simulink model "Crane_LQR_disc_Kalman"  (R2018a)
settings: Solver=VariableStepAuto  StartTime=0.0  StopTime=30  RelTol=1e-3
undefined symbols (not defined in the file): A, B, C, D, Discrete, F, L, sigbuilder_block, Time, Ts, xinit
libraries: dspsrcs4 x1, ctrlSharedLib x1
settings Model: Creator=tcbooij  LastModifiedBy=TU Delf SID
settings CodeAppCC: StateflowObjectComments=on

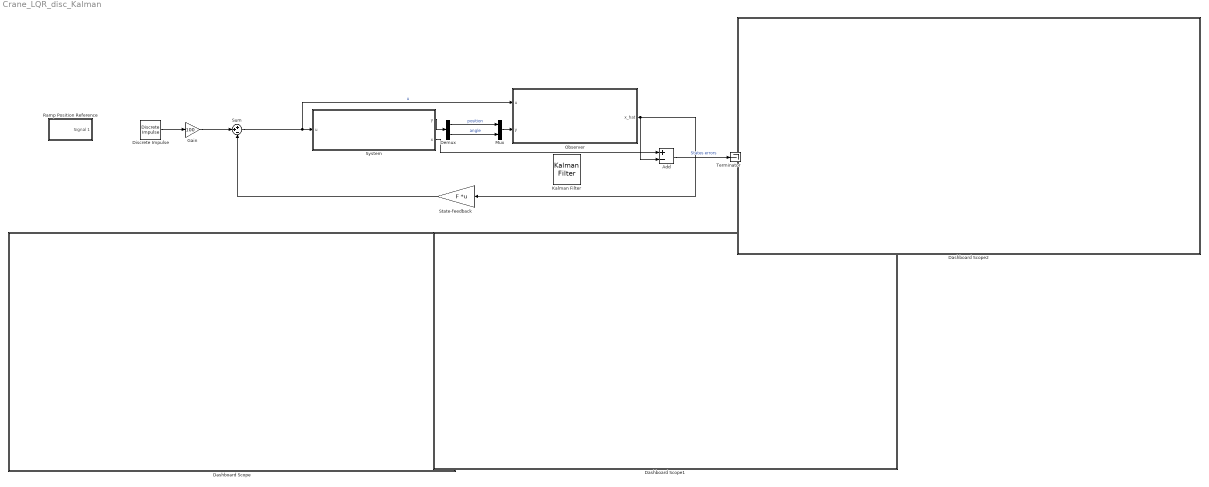
== system Crane_LQR_disc_Kalman ==
  Add : Sum  Inputs=+-
  Dashboard Scope : Subsystem  DialogController=hmiCreateDDGDialog  IsWebBlock=on  mask(MWDashboardBlock){webBlockId=2d634a0c-9c30-41ca-882d-9c1a5de680b0, webBlockType=sdiscope, ShowInitialText=on, HMISrcModelName=Crane_LQR_disc2}
      mask prompts: webBlockId "WebBlock Id"; webBlockType "WebBlock Type"; HMISrcModelName "Source Model"
      mask help: SimulinkHMI:dialogs:HMIScopeDialogDesc
      mask Help: helpview([docroot '/mapfiles/simulink.map'], 'hmi_scope')
      mask Display:
      | if strcmp(get_param(bdroot(gcb),'BlockDiagramType'), 'library')
      |     image([(matlabroot) '/toolbox/simulink/hmi/icons/DashboardScope.png']);
      | end
  Dashboard Scope1 : Subsystem  DialogController=hmiCreateDDGDialog  IsWebBlock=on  mask(MWDashboardBlock){webBlockId=94ce42f8-c4e1-41da-82c1-a31c02963333, webBlockType=sdiscope, ShowInitialText=on, HMISrcModelName=Crane_LQR_disc2}
      mask prompts: webBlockId "WebBlock Id"; webBlockType "WebBlock Type"; HMISrcModelName "Source Model"
      mask help: SimulinkHMI:dialogs:HMIScopeDialogDesc
      mask Help: helpview([docroot '/mapfiles/simulink.map'], 'hmi_scope')
      mask Display:
      | if strcmp(get_param(bdroot(gcb),'BlockDiagramType'), 'library')
      |     image([(matlabroot) '/toolbox/simulink/hmi/icons/DashboardScope.png']);
      | end
  Dashboard Scope2 : Subsystem  DialogController=hmiCreateDDGDialog  IsWebBlock=on  mask(MWDashboardBlock){webBlockId=eee89b98-8c9a-4aeb-b6f7-67e202be8cd2, webBlockType=sdiscope, ShowInitialText=on, HMISrcModelName=Crane_LQR_disc2}
      mask prompts: webBlockId "WebBlock Id"; webBlockType "WebBlock Type"; HMISrcModelName "Source Model"
      mask help: SimulinkHMI:dialogs:HMIScopeDialogDesc
      mask Help: helpview([docroot '/mapfiles/simulink.map'], 'hmi_scope')
      mask Display:
      | if strcmp(get_param(bdroot(gcb),'BlockDiagramType'), 'library')
      |     image([(matlabroot) '/toolbox/simulink/hmi/icons/DashboardScope.png']);
      | end
  Demux : Demux  Outputs=2
  Discrete Impulse : dspsrcs4/Discrete  Impulse  Delay=200  SampleTime=0.01  FrameSample=1  OutputFrames=off  dataType=double  isSigned=on  wordLen=16  udDataType=sfix(16)  fracBitsMode=Best precision  numFracBits=15  OutDataTypeStr=double  LastOutDataTypeStr=double
  Gain : Gain  Gain=100
  Kalman Filter : ctrlSharedLib/Kalman Filter  TimeDomain=Discrete-Time  UseCurrentEstimator=on  ModelSource=Individual A, B, C, D matrices  ModelSourceVariable=ss(A,B,C,D,Ts)  A=A  B=B  C=C  D=D  NumberOfStates=1  NumberOfInputs=1  NumberOfOutputs=1  InitialEstimateSource=Dialog  X0=0  P0=10  UseK=off  UseGH=off  NumberOfProcessNoiseInputs=1  G=1  TimeInvariantG=on  H=0  TimeInvariantH=on  Q=0.05  TimeInvariantQ=on  R=1  TimeInvariantR=on  N=0  TimeInvariantN=on  AddInputPort=on  AddEnablePort=off  OutputEstimatedY=off  OutputP=off  Ts=-1
      settings: SourceProductBaseCode=CT
  Mux : Mux  Inputs=2
  Observer : Subsystem
  Ramp Position Reference : Subsystem  Tag=STV Subsys  LoadFcn=sigbuilder_block('load');  StartFcn=sigbuilder_block('start');  StopFcn=sigbuilder_block('stop');  ClipboardFcn=sigbuilder_block('clipboard');  mask(Sigbuilder block){tuvar=[0:10]}
      mask help: Simulink:masks:SigbuilderBlock_MD
      mask init:
      | if ~strcmp(get_param(bdroot(gcbh),'SimulationStatus'),'stopped') tuvar = sigbuilder_block('maskInit'); end
      settings: CopyFcn=sigbuilder_block('copy');  DeleteFcn=sigbuilder_block('delete');  ModelCloseFcn=sigbuilder_block('modelClose');  PreSaveFcn=sigbuilder_block('preSave');  PauseFcn=sigbuilder_block('pause');  ContinueFcn=sigbuilder_block('continue');  NameChangeFcn=sigbuilder_block('namechange');  OpenFcn=sigbuilder_block('open',[294 84 558 400.5 ]);  CloseFcn=sigbuilder_block('close');
      mask Display: plot(0, 0, 100, 100,[2, 2, 32, 32, 2], [68, 8, 8, 68, 68],[32, 2], [38, 38], [32, 19, 2],[53, 60, 44], [32, 17, 17, 2],[16, 16, 31, 31]);txt = getActiveGroup(gcbh);text(2, 100, txt,'verticalAlignment', 'top');
  State-feedback : Gain  Gain=F  Multiplication=Matrix(K*u)
  Sum : Sum  Inputs=++-
  System : Subsystem
  Terminator : Terminator
  wires:
  Sum/1 -> Observer/1(u), System/1(u)  "u"
  State-feedback/1 -> Sum/3
  Observer/1(x_hat) -> Add/2, State-feedback/1
  System/1(y) -> Demux/1
  Mux/1 -> Observer/2(y)
  Demux/1 -> Mux/1  "position"
  Demux/2 -> Mux/2  "angle"
  Discrete Impulse/1 -> Gain/1
  Gain/1 -> Sum/2
  System/2(x) -> Add/1
  Add/1 -> Terminator/1  "States errors"

== system Crane_LQR_disc_Kalman/Dashboard Scope ==

== system Crane_LQR_disc_Kalman/Dashboard Scope1 ==

== system Crane_LQR_disc_Kalman/Dashboard Scope2 ==

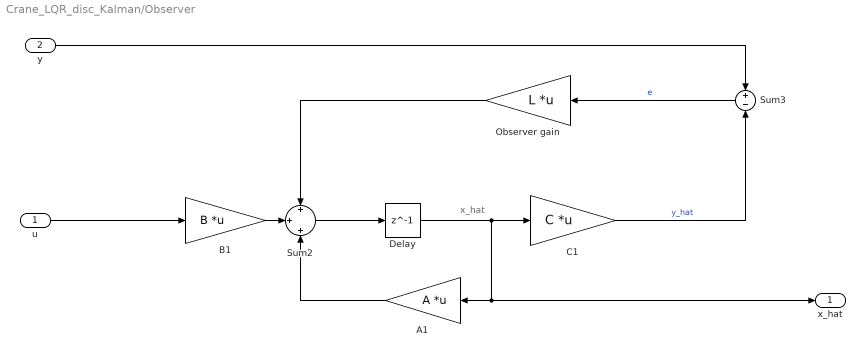
== system Crane_LQR_disc_Kalman/Observer ==
  note: x_hat
  u : Inport
  y : Inport  Port=2
  A1 : Gain  Gain=A  Multiplication=Matrix(K*u)
  B1 : Gain  Gain=B  Multiplication=Matrix(K*u)
  C1 : Gain  Gain=C  Multiplication=Matrix(K*u)
  Delay : Delay  DelayLength=1
  Observer gain : Gain  Gain=L  Multiplication=Matrix(K*u)
  Sum2 : Sum  Inputs=+|+|+
  Sum3 : Sum  Inputs=+|-
  x_hat : Outport
  wires:
  Sum3/1 -> Observer gain/1  "e"
  y/1 -> Sum3/1
  A1/1 -> Sum2/3
  B1/1 -> Sum2/2
  u/1 -> B1/1
  C1/1 -> Sum3/2  "y_hat"
  Observer gain/1 -> Sum2/1
  Delay/1 -> x_hat/1, A1/1, C1/1
  Sum2/1 -> Delay/1

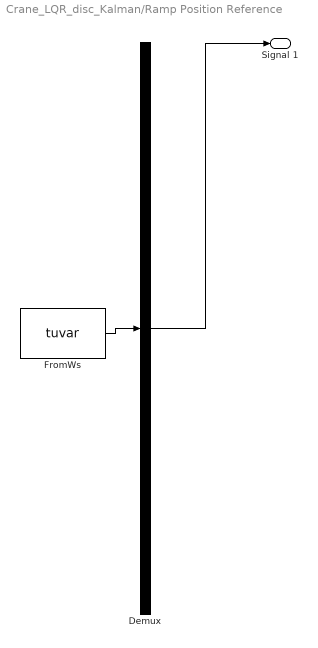
== system Crane_LQR_disc_Kalman/Ramp Position Reference ==
  Demux : Demux  Tag=STV Demux  Outputs=1
  FromWs : FromWorkspace  Tag=STV FromWs  VariableName=tuvar  SampleTime=0
      SigBuilderData=|
      | common.afterFinalStr = 'Extrapolate'
      | common.sampleTime = 0
      | dataSet.timeRange = [0 30]
      | dataSet.name = 'Group 1'
      | sbobj.Groups.Name = 'Group 1'
      | sbobj.Groups.Signals.Name = 'Signal 1'
      | sbobj.Groups.Signals.XData = [0 4 6 10 30]
      | sbobj.Groups.Signals.YData = [0 1 1 1.005 1.005]
      | sbobj.Groups.TimeRange = [0 30]
  Signal 1 : Outport  Tag=STV Outport
  wires:
  Demux/1 -> Signal 1/1
  FromWs/1 -> Demux/1

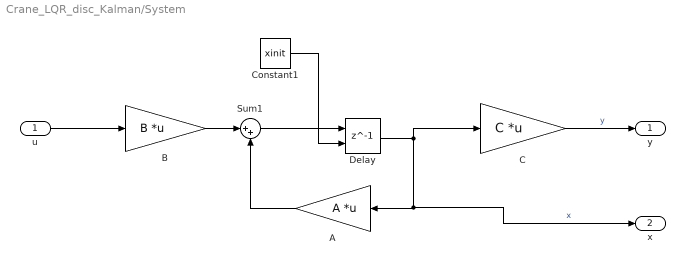
== system Crane_LQR_disc_Kalman/System ==
  u : Inport
  A : Gain  Gain=A  Multiplication=Matrix(K*u)
  B : Gain  Gain=B  Multiplication=Matrix(K*u)
  C : Gain  Gain=C  Multiplication=Matrix(K*u)
  Constant1 : Constant  Value=xinit
  Delay : Delay  DelayLength=1  InitialConditionSource=Input port
      settings: InputPortMap=u0,p4
  Sum1 : Sum  Inputs=|++
  y : Outport
  x : Outport  Port=2
  wires:
  Sum1/1 -> Delay/1
  u/1 -> B/1
  C/1 -> y/1  "y"
  Delay/1 -> C/1, x/1, A/1  "x"
  A/1 -> Sum1/2
  B/1 -> Sum1/1
  Constant1/1 -> Delay/2
